simulink library "MotorModelLapSL"  (R2016b)
settings: Solver=VariableStepAuto  StartTime=0.0  StopTime=10.0  RelTol=1e-3
undefined symbols (not defined in the file): CAL_B_NmPerW, CAL_flux_e, CAL_Inertia_J, CAL_Re_ohm, CAL_SimInduct_H
settings Model: Creator=oelkawok  LastModifiedBy=oelkawok

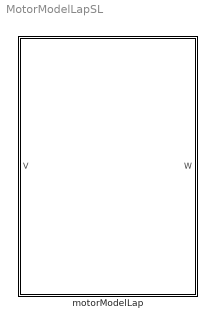
== system MotorModelLapSL ==
  motorModelLap : Subsystem

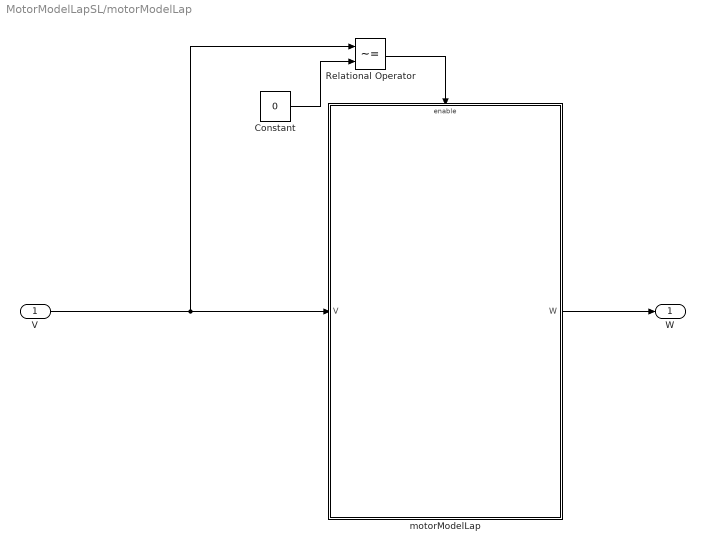
== system MotorModelLapSL/motorModelLap ==
  V : Inport
  Constant : Constant  Value=0
  Relational Operator : RelationalOperator  Operator=~=  OutDataTypeStr=boolean  RndMeth=Simplest
  motorModelLap : Subsystem
  W : Outport  OutputWhenDisabled=reset  InitialOutput=0
  wires:
  motorModelLap/1(W) -> W/1
  V/1 -> Relational Operator/1, motorModelLap/1(V)
  Relational Operator/1 -> motorModelLap/Enable
  Constant/1 -> Relational Operator/2

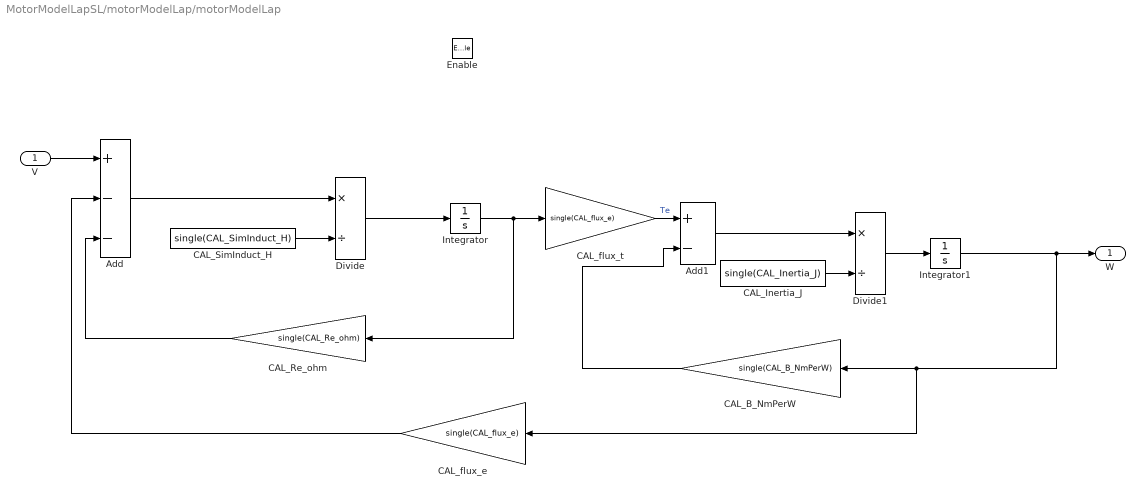
== system MotorModelLapSL/motorModelLap/motorModelLap ==
  V : Inport
  Enable : EnablePort  StatesWhenEnabling=reset
  Add : Sum  Inputs=+--
  Add1 : Sum  Inputs=+-
  CAL_B_NmPerW : Gain  Gain=single(CAL_B_NmPerW)
  CAL_Inertia_J : Constant  Value=single(CAL_Inertia_J)
  CAL_Re_ohm : Gain  Gain=single(CAL_Re_ohm)
  CAL_SimInduct_H : Constant  Value=single(CAL_SimInduct_H)
  CAL_flux_e : Gain  Gain=single(CAL_flux_e)
  CAL_flux_t : Gain  Gain=single(CAL_flux_e)
  Divide : Product  Inputs=*/
  Divide1 : Product  Inputs=*/
  Integrator : Integrator
  Integrator1 : Integrator
  W : Outport  OutputWhenDisabled=reset  InitialOutput=0
  wires:
  Integrator/1 -> CAL_Re_ohm/1, CAL_flux_t/1
  V/1 -> Add/1
  Integrator1/1 -> CAL_B_NmPerW/1, CAL_flux_e/1, W/1
  CAL_Re_ohm/1 -> Add/3
  Divide1/1 -> Integrator1/1
  CAL_SimInduct_H/1 -> Divide/2
  CAL_Inertia_J/1 -> Divide1/2
  CAL_flux_t/1 -> Add1/1  "Te"
  CAL_flux_e/1 -> Add/2
  Add1/1 -> Divide1/1
  CAL_B_NmPerW/1 -> Add1/2
  Divide/1 -> Integrator/1
  Add/1 -> Divide/1
